simulink model "Robot"  (R2022b)
settings: Solver=FixedStepDiscrete  StartTime=0.0  StopTime=30  FixedStep=0.001  RelTol=1e-3
InitFcn:
  | load("BusConfig.mat");
undefined symbols (not defined in the file or in its folder): DiscIntNeverNeededParam
libraries: slrealtimeethercatlib x119, simulink x20
(part 3 of 7)

== system Robot/Motor2 Torque Control Init Frame/State_2_Enable ==
  State : Inport
  Subsystem : Subsystem
  Switch Case : SwitchCase  CaseConditions={TaskIndex}
  Enable : Outport
  FinishIndex : Outport  Port=2
  wires:
  Switch Case/2 -> Subsystem/2(Case Default)
  Switch Case/1 -> Subsystem/1(Case)
  Subsystem/2(FinishIndex) -> FinishIndex/1
  Subsystem/1(Enable) -> Enable/1
  State/1 -> Switch Case/1

== system Robot/Motor2 Torque Control Init Frame/State_3_Enable ==
  State : Inport
  Subsystem : Subsystem
  Switch Case : SwitchCase  CaseConditions={TaskIndex}
  Enable : Outport
  FinishIndex : Outport  Port=2
  wires:
  Switch Case/2 -> Subsystem/2(Case Default)
  Switch Case/1 -> Subsystem/1(Case)
  Subsystem/2(FinishIndex) -> FinishIndex/1
  Subsystem/1(Enable) -> Enable/1
  State/1 -> Switch Case/1

== system Robot/Motor2 Torque Control Init Frame/State_4_Enable ==
  State : Inport
  Subsystem : Subsystem
  Switch Case : SwitchCase  CaseConditions={TaskIndex}
  Enable : Outport
  FinishIndex : Outport  Port=2
  wires:
  Switch Case/2 -> Subsystem/2(Case Default)
  Switch Case/1 -> Subsystem/1(Case)
  Subsystem/2(FinishIndex) -> FinishIndex/1
  Subsystem/1(Enable) -> Enable/1
  State/1 -> Switch Case/1

== system Robot/Motor2 Torque Control Init Frame/State_5_Enable ==
  State : Inport
  Subsystem : Subsystem
  Switch Case : SwitchCase  CaseConditions={TaskIndex}
  Enable : Outport
  FinishIndex : Outport  Port=2
  wires:
  Switch Case/2 -> Subsystem/2(Case Default)
  Switch Case/1 -> Subsystem/1(Case)
  Subsystem/2(FinishIndex) -> FinishIndex/1
  Subsystem/1(Enable) -> Enable/1
  State/1 -> Switch Case/1

== system Robot/Motor2 Torque Control Init Frame/State_6_Enable ==
  State : Inport
  Subsystem : Subsystem
  Switch Case : SwitchCase  CaseConditions={TaskIndex}
  Enable : Outport
  FinishIndex : Outport  Port=2
  wires:
  Switch Case/2 -> Subsystem/2(Case Default)
  Switch Case/1 -> Subsystem/1(Case)
  Subsystem/2(FinishIndex) -> FinishIndex/1
  Subsystem/1(Enable) -> Enable/1
  State/1 -> Switch Case/1

== system Robot/Motor2 Torque Control Init Frame/State_7_Enable ==
  State : Inport
  Subsystem : Subsystem
  Switch Case : SwitchCase  CaseConditions={TaskIndex}
  Enable : Outport
  FinishIndex : Outport  Port=2
  wires:
  Switch Case/2 -> Subsystem/2(Case Default)
  Switch Case/1 -> Subsystem/1(Case)
  Subsystem/2(FinishIndex) -> FinishIndex/1
  Subsystem/1(Enable) -> Enable/1
  State/1 -> Switch Case/1

== system Robot/Motor2 Torque Control Init Frame/State_8_Enable ==
  State : Inport
  Subsystem : Subsystem
  Switch Case : SwitchCase  CaseConditions={TaskIndex}
  Enable : Outport
  FinishIndex : Outport  Port=2
  wires:
  Switch Case/2 -> Subsystem/2(Case Default)
  Switch Case/1 -> Subsystem/1(Case)
  Subsystem/2(FinishIndex) -> FinishIndex/1
  Subsystem/1(Enable) -> Enable/1
  State/1 -> Switch Case/1

== system Robot/Motor2 Torque Control Init Frame/State_9_Enable ==
  State : Inport
  Subsystem : Subsystem
  Switch Case : SwitchCase  CaseConditions={TaskIndex}
  Enable : Outport
  FinishIndex : Outport  Port=2
  wires:
  Switch Case/2 -> Subsystem/2(Case Default)
  Switch Case/1 -> Subsystem/1(Case)
  Subsystem/2(FinishIndex) -> FinishIndex/1
  Subsystem/1(Enable) -> Enable/1
  State/1 -> Switch Case/1

== system Robot/Motor3 Torque Control Init Frame/Get MasterState OP Frame ==
  FinishIndex : Inport
  Enable : EnablePort
  Clock : Clock
  Constant4 : Constant  Value=0  OutDataTypeStr=double
  Constant5 : Constant
  Display{1,3..5} (4 alike) : Display
  EtherCAT PDO Receive1 : slrealtimeethercatlib/EtherCAT PDO Receive  Priority=2  sig_name=Drive 3 (Elmo Drive ).Inputs.Status word  sig_offset=24832  sig_type=uint16  type_size=16  sig_dim=1  device_id=0  sample_time=0.001000
  Get Device State : slrealtimeethercatlib/Get Device State  device_id=0  slave_name=Drive 3 (Elmo Drive )  sample_time=0.001  slave_addr=1003  selected_slave=Term 1 (EK1100)  timeout=500  slave_found=1
  If Action Subsystem5 : Subsystem  TreatAsAtomicUnit=on
  If Action Subsystem6 : Subsystem  TreatAsAtomicUnit=on
  If Action Subsystem7 : Subsystem  TreatAsAtomicUnit=on
  If1 : If  IfExpression=(u1 == 4663)
  If2 : If  IfExpression=(u1 == 8)
  Merge1 : Merge
  TaskFinished : Outport
  wires:
  If Action Subsystem6/1(Out1) -> Merge1/2
  EtherCAT PDO Receive1/1 -> Display3/1
  Get Device State/1 -> If2/1, Display1/1
  If Action Subsystem7/1(Out1) -> Display5/1
  If Action Subsystem5/1(Out1) -> Merge1/1
  Constant4/1 -> If Action Subsystem6/1(In1)
  Merge1/1 -> TaskFinished/1
  If1/1 -> If Action Subsystem7/Action
  Constant5/1 -> If Action Subsystem7/1(In1)
  If2/1 -> If Action Subsystem5/Action
  If2/2 -> If Action Subsystem6/Action
  Clock/1 -> Display4/1
  FinishIndex/1 -> If Action Subsystem5/1(In1)

== system Robot/Motor3 Torque Control Init Frame/PDO Set 0x6040:6->7->15 Frame ==
  FinishIndex : Inport
  Enable : EnablePort
  Clock : Clock
  Constant : Constant  Value=6  OutDataTypeStr=uint16
  Constant1 : Constant  Value=7  OutDataTypeStr=uint16
  Constant2 : Constant  Value=15  OutDataTypeStr=uint16
  Constant4 : Constant  Value=0  OutDataTypeStr=double
  Constant5 : Constant
  Counter Limited : simulink/Sources/Counter Limited  uplimit=500  tsamp=-1
  Display{1..5} (5 alike) : Display
  EtherCAT PDO Receive1 : slrealtimeethercatlib/EtherCAT PDO Receive  Priority=2  sig_name=Drive 3 (Elmo Drive ).Inputs.Status word  sig_offset=24832  sig_type=uint16  type_size=16  sig_dim=1  device_id=0  sample_time=0.001000
  EtherCAT PDO Transmit1 : slrealtimeethercatlib/EtherCAT PDO Transmit  Priority=3  sig_name=Drive 3 (Elmo Drive ).Outputs.Control word  sig_offset=24800  sig_type=uint16  type_size=16  sig_dim=1  device_id=0  sample_time=0.001000
  If : If  NumInputs=2  IfExpression=(u1 == 720)&(u2 == 500)  ElseIfExpressions=(u1 == 689)&(u2 == 500), (u1 == 691)&(u2 == 500)
  If Action Subsystem : Subsystem  TreatAsAtomicUnit=on
  If Action Subsystem1 : Subsystem  TreatAsAtomicUnit=on
  If Action Subsystem2 : Subsystem  TreatAsAtomicUnit=on
  If Action Subsystem4 : Subsystem  TreatAsAtomicUnit=on
  If Action Subsystem5 : Subsystem  TreatAsAtomicUnit=on
  If Action Subsystem6 : Subsystem  TreatAsAtomicUnit=on
  If Action Subsystem7 : Subsystem  TreatAsAtomicUnit=on
  If1 : If  IfExpression=(u1 == 4663)|(u1 == 4791)
  If2 : If  IfExpression=(u1 >= 0.1)
  Memory : Memory
  Merge : Merge  Inputs=4
  Merge1 : Merge
  TaskFinished : Outport
  wires:
  If Action Subsystem2/1(Out1) -> Merge/3
  If Action Subsystem7/1(Out1) -> If2/1, Display5/1
  If Action Subsystem6/1(Out1) -> Merge1/2
  EtherCAT PDO Receive1/1 -> If1/1, If/1, Display1/1
  If/2 -> If Action Subsystem1/Action
  Memory/1 -> If Action Subsystem4/1(In1)
  Constant5/1 -> If Action Subsystem7/1(In1)
  Constant1/1 -> If Action Subsystem1/1(In1)
  Constant/1 -> If Action Subsystem/1(In1)
  If Action Subsystem1/1(Out1) -> Merge/2
  If/4 -> If Action Subsystem4/Action
  Constant2/1 -> If Action Subsystem2/1(In1)
  If/3 -> If Action Subsystem2/Action
  If/1 -> If Action Subsystem/Action
  Clock/1 -> Display4/1
  If1/1 -> If Action Subsystem7/Action
  If2/1 -> If Action Subsystem5/Action
  Merge/1 -> Display2/1, EtherCAT PDO Transmit1/1, Memory/1
  Merge1/1 -> TaskFinished/1
  FinishIndex/1 -> If Action Subsystem5/1(In1)
  If2/2 -> If Action Subsystem6/Action
  If Action Subsystem4/1(Out1) -> Merge/4
  Counter Limited/1 -> If/2, Display3/1
  Constant4/1 -> If Action Subsystem6/1(In1)
  If Action Subsystem5/1(Out1) -> Merge1/1
  If Action Subsystem/1(Out1) -> Merge/1

== system Robot/Motor3 Torque Control Init Frame/SDO Get 0x6075 Frame ==
  FinishIndex : Inport
  Enable : EnablePort
  Clock : Clock
  Constant : Constant  OutDataTypeStr=int32
  Constant4 : Constant  Value=0  OutDataTypeStr=double
  Constant5 : Constant
  Display{,1,3..5} (5 alike) : Display
  EtherCAT Async SDO Upload : slrealtimeethercatlib/EtherCAT Async SDO Upload  index=0x6075  subIndex=0  sig_type=uint32  sig_dim=1  device_id=0  slave_name=Drive 3 (Elmo Drive )  sample_time=-1  slave_addr=1003  selected_slave=Term 1 (EK1100)  timeout=3000  slave_found=1  complete=0
  If Action Subsystem5 : Subsystem  TreatAsAtomicUnit=on
  If Action Subsystem6 : Subsystem  TreatAsAtomicUnit=on
  If Action Subsystem7 : Subsystem  TreatAsAtomicUnit=on
  If1 : If  IfExpression=(u1 == 4663)
  If2 : If  IfExpression=(u1 == 2)
  Merge1 : Merge
  TaskFinished : Outport
  RatedCurrent : Outport  Port=2
  wires:
  EtherCAT Async SDO Upload/1 -> RatedCurrent/1, Display/1
  EtherCAT Async SDO Upload/3 -> Display3/1
  EtherCAT Async SDO Upload/2 -> If2/1, Display1/1
  Constant/1 -> EtherCAT Async SDO Upload/1
  If2/1 -> If Action Subsystem5/Action
  Merge1/1 -> TaskFinished/1
  Clock/1 -> Display4/1
  If2/2 -> If Action Subsystem6/Action
  If Action Subsystem7/1(Out1) -> Display5/1
  Constant4/1 -> If Action Subsystem6/1(In1)
  If1/1 -> If Action Subsystem7/Action
  If Action Subsystem5/1(Out1) -> Merge1/1
  If Action Subsystem6/1(Out1) -> Merge1/2
  Constant5/1 -> If Action Subsystem7/1(In1)
  FinishIndex/1 -> If Action Subsystem5/1(In1)

== system Robot/Motor3 Torque Control Init Frame/SDO Set 0x6040:15 Frame ==
  FinishIndex : Inport
  Enable : EnablePort
  Bitwise Operator : simulink/Logic and Bit Operations/Bitwise Operator  logicop=AND  UseBitMask=on  BitMask=bin2dec('0000000000000111')  BitMaskRealWorld=Stored Integer
  Clock : Clock
  Constant : Constant  Value=15  OutDataTypeStr=uint16
  Constant1 : Constant  OutDataTypeStr=int32
  Constant2 : Constant  Value=0  OutDataTypeStr=int32
  Constant4 : Constant  Value=0  OutDataTypeStr=double
  Constant5 : Constant
  Constant6 : Constant  OutDataTypeStr=int32
  Constant7 : Constant
  Constant8 : Constant  Value=0b0000000000000111  OutDataTypeStr=uint16
  Display{1..6} (6 alike) : Display
  EtherCAT Async SDO Download : slrealtimeethercatlib/EtherCAT Async SDO Download  index=0x6040  subIndex=0  sig_type=uint16  sig_dim=1  device_id=0  slave_name=Drive 3 (Elmo Drive )  sample_time=-1  slave_addr=1003  selected_slave=Term 1 (EK1100)  timeout=2000  slave_found=1  complete=0
  EtherCAT PDO Receive1 : slrealtimeethercatlib/EtherCAT PDO Receive  Priority=2  sig_name=Drive 4 (Elmo Drive ).Inputs.Status word  sig_offset=39136  sig_type=uint16  type_size=16  sig_dim=1  device_id=0  sample_time=0.001
  If Action Subsystem1 : Subsystem  TreatAsAtomicUnit=on
  If Action Subsystem2 : Subsystem  TreatAsAtomicUnit=on
  If Action Subsystem3 : Subsystem  TreatAsAtomicUnit=on
  If Action Subsystem5 : Subsystem  TreatAsAtomicUnit=on
  If Action Subsystem6 : Subsystem  TreatAsAtomicUnit=on
  If Action Subsystem7 : Subsystem  TreatAsAtomicUnit=on
  If1 : If  IfExpression=(u1 == 4663)
  If2 : If  IfExpression=(u1 == 2)
  If3 : If  NumInputs=2  IfExpression=(u1 == u2)
  If4 : If  IfExpression=(u1 >= 0.1)
  Merge1 : Merge
  Merge2 : Merge
  TaskFinished : Outport
  wires:
  Constant8/1 -> If3/2
  Bitwise Operator/1 -> If3/1
  If Action Subsystem3/1(Out1) -> Display6/1, If4/1
  Clock/1 -> Display4/1
  Merge1/1 -> TaskFinished/1
  If Action Subsystem2/1(Out1) -> Merge2/2
  If Action Subsystem1/1(Out1) -> Merge2/1
  Constant7/1 -> If Action Subsystem3/1(In1)
  If2/2 -> If Action Subsystem6/Action
  EtherCAT PDO Receive1/1 -> Display3/1, Bitwise Operator/1
  If3/1 -> If Action Subsystem3/Action
  If4/1 -> If Action Subsystem1/Action
  Constant6/1 -> If Action Subsystem2/1(In1)
  If4/2 -> If Action Subsystem2/Action
  EtherCAT Async SDO Download/1 -> If2/1, Display1/1
  Constant4/1 -> If Action Subsystem6/1(In1)
  Constant5/1 -> If Action Subsystem7/1(In1)
  Constant1/1 -> EtherCAT Async SDO Download/2
  If Action Subsystem6/1(Out1) -> Merge1/2
  If Action Subsystem7/1(Out1) -> Display5/1
  If2/1 -> If Action Subsystem5/Action
  Constant2/1 -> If Action Subsystem1/1(In1)
  If1/1 -> If Action Subsystem7/Action
  FinishIndex/1 -> If Action Subsystem5/1(In1)
  EtherCAT Async SDO Download/2 -> Display2/1
  Constant/1 -> EtherCAT Async SDO Download/1
  If Action Subsystem5/1(Out1) -> Merge1/1

== system Robot/Motor3 Torque Control Init Frame/SDO Set 0x6040:31 Frame ==
  FinishIndex : Inport
  Enable : EnablePort
  Bitwise Operator : simulink/Logic and Bit Operations/Bitwise Operator  logicop=AND  UseBitMask=on  BitMask=bin2dec('0001010000010111')  BitMaskRealWorld=Stored Integer
  Clock : Clock
  Constant : Constant  Value=31  OutDataTypeStr=uint16
  Constant1 : Constant  OutDataTypeStr=int32
  Constant2 : Constant  Value=0  OutDataTypeStr=int32
  Constant4 : Constant  Value=0  OutDataTypeStr=double
  Constant5 : Constant
  Constant6 : Constant  OutDataTypeStr=int32
  Constant7 : Constant
  Constant8 : Constant  Value=0b0001010000010111  OutDataTypeStr=uint16
  Display{1..6} (6 alike) : Display
  EtherCAT Async SDO Download : slrealtimeethercatlib/EtherCAT Async SDO Download  index=0x6040  subIndex=0  sig_type=uint16  sig_dim=1  device_id=0  slave_name=Drive 3 (Elmo Drive )  sample_time=-1  slave_addr=1003  selected_slave=Term 1 (EK1100)  timeout=2000  slave_found=1  complete=0
  EtherCAT PDO Receive1 : slrealtimeethercatlib/EtherCAT PDO Receive  Priority=2  sig_name=Drive 3 (Elmo Drive ).Inputs.Status word  sig_offset=24832  sig_type=uint16  type_size=16  sig_dim=1  device_id=0  sample_time=0.001
  If Action Subsystem1 : Subsystem  TreatAsAtomicUnit=on
  If Action Subsystem2 : Subsystem  TreatAsAtomicUnit=on
  If Action Subsystem3 : Subsystem  TreatAsAtomicUnit=on
  If Action Subsystem5 : Subsystem  TreatAsAtomicUnit=on
  If Action Subsystem6 : Subsystem  TreatAsAtomicUnit=on
  If Action Subsystem7 : Subsystem  TreatAsAtomicUnit=on
  If1 : If  IfExpression=(u1 == 4663)
  If2 : If  IfExpression=(u1 == 2)
  If3 : If  NumInputs=2  IfExpression=(u1 == u2)
  If4 : If  IfExpression=(u1 >= 0.1)
  Merge1 : Merge
  Merge2 : Merge
  TaskFinished : Outport
  wires:
  If1/1 -> If Action Subsystem7/Action
  If Action Subsystem5/1(Out1) -> Merge1/1
  If Action Subsystem6/1(Out1) -> Merge1/2
  FinishIndex/1 -> If Action Subsystem5/1(In1)
  If2/1 -> If Action Subsystem5/Action
  If4/2 -> If Action Subsystem2/Action
  EtherCAT Async SDO Download/1 -> If2/1, Display1/1
  Constant/1 -> EtherCAT Async SDO Download/1
  Bitwise Operator/1 -> If3/1
  If Action Subsystem7/1(Out1) -> Display5/1
  Constant8/1 -> If3/2
  If2/2 -> If Action Subsystem6/Action
  If Action Subsystem3/1(Out1) -> Display6/1, If4/1
  If Action Subsystem2/1(Out1) -> Merge2/2
  If3/1 -> If Action Subsystem3/Action
  Constant4/1 -> If Action Subsystem6/1(In1)
  Constant6/1 -> If Action Subsystem2/1(In1)
  If4/1 -> If Action Subsystem1/Action
  Constant1/1 -> EtherCAT Async SDO Download/2
  EtherCAT PDO Receive1/1 -> Display3/1, Bitwise Operator/1
  Clock/1 -> Display4/1
  If Action Subsystem1/1(Out1) -> Merge2/1
  Merge1/1 -> TaskFinished/1
  Constant2/1 -> If Action Subsystem1/1(In1)
  EtherCAT Async SDO Download/2 -> Display2/1
  Constant5/1 -> If Action Subsystem7/1(In1)
  Constant7/1 -> If Action Subsystem3/1(In1)

== system Robot/Motor3 Torque Control Init Frame/SDO Set 0x6040:6 Frame ==
  FinishIndex : Inport
  Enable : EnablePort
  Bitwise Operator : simulink/Logic and Bit Operations/Bitwise Operator  logicop=AND  UseBitMask=on  BitMask=bin2dec('0000000000000001')  BitMaskRealWorld=Stored Integer
  Clock : Clock
  Constant : Constant  Value=6  OutDataTypeStr=uint16
  Constant1 : Constant  OutDataTypeStr=int32
  Constant2 : Constant  Value=0  OutDataTypeStr=int32
  Constant4 : Constant  Value=0  OutDataTypeStr=double
  Constant5 : Constant
  Constant6 : Constant  OutDataTypeStr=int32
  Constant7 : Constant
  Constant8 : Constant  Value=0b0000000000000001  OutDataTypeStr=uint16
  Display{1..6} (6 alike) : Display
  EtherCAT Async SDO Download : slrealtimeethercatlib/EtherCAT Async SDO Download  index=0x6040  subIndex=0  sig_type=uint16  sig_dim=1  device_id=0  slave_name=Drive 3 (Elmo Drive )  sample_time=-1  slave_addr=1003  selected_slave=Term 1 (EK1100)  timeout=3000  slave_found=1  complete=0
  EtherCAT PDO Receive1 : slrealtimeethercatlib/EtherCAT PDO Receive  Priority=2  sig_name=Drive 3 (Elmo Drive ).Inputs.Status word  sig_offset=24832  sig_type=uint16  type_size=16  sig_dim=1  device_id=0  sample_time=0.001
  If Action Subsystem1 : Subsystem  TreatAsAtomicUnit=on
  If Action Subsystem2 : Subsystem  TreatAsAtomicUnit=on
  If Action Subsystem3 : Subsystem  TreatAsAtomicUnit=on
  If Action Subsystem5 : Subsystem  TreatAsAtomicUnit=on
  If Action Subsystem6 : Subsystem  TreatAsAtomicUnit=on
  If Action Subsystem7 : Subsystem  TreatAsAtomicUnit=on
  If1 : If  IfExpression=(u1 == 4663)
  If2 : If  IfExpression=(u1 == 2)
  If3 : If  NumInputs=2  IfExpression=(u1 == u2)
  If4 : If  IfExpression=(u1 >= 0.1)
  Merge1 : Merge
  Merge2 : Merge
  TaskFinished : Outport
  wires:
  Constant2/1 -> If Action Subsystem1/1(In1)
  Constant/1 -> EtherCAT Async SDO Download/1
  If1/1 -> If Action Subsystem7/Action
  Constant4/1 -> If Action Subsystem6/1(In1)
  If4/1 -> If Action Subsystem1/Action
  If Action Subsystem1/1(Out1) -> Merge2/1
  If2/2 -> If Action Subsystem6/Action
  Bitwise Operator/1 -> If3/1
  FinishIndex/1 -> If Action Subsystem5/1(In1)
  EtherCAT Async SDO Download/2 -> Display2/1
  EtherCAT Async SDO Download/1 -> If2/1, Display1/1
  If2/1 -> If Action Subsystem5/Action
  If4/2 -> If Action Subsystem2/Action
  Constant5/1 -> If Action Subsystem7/1(In1)
  If Action Subsystem2/1(Out1) -> Merge2/2
  Constant7/1 -> If Action Subsystem3/1(In1)
  If Action Subsystem3/1(Out1) -> Display6/1, If4/1
  If Action Subsystem5/1(Out1) -> Merge1/1
  Constant6/1 -> If Action Subsystem2/1(In1)
  If Action Subsystem6/1(Out1) -> Merge1/2
  Constant1/1 -> EtherCAT Async SDO Download/2
  If3/1 -> If Action Subsystem3/Action
  If Action Subsystem7/1(Out1) -> Display5/1
  Constant8/1 -> If3/2
  EtherCAT PDO Receive1/1 -> Display3/1, Bitwise Operator/1
  Clock/1 -> Display4/1
  Merge1/1 -> TaskFinished/1

== system Robot/Motor3 Torque Control Init Frame/SDO Set 0x6040:7 Frame ==
  FinishIndex : Inport
  Enable : EnablePort
  Bitwise Operator : simulink/Logic and Bit Operations/Bitwise Operator  logicop=AND  UseBitMask=on  BitMask=bin2dec('0000000000000011')  BitMaskRealWorld=Stored Integer
  Clock : Clock
  Constant : Constant  Value=7  OutDataTypeStr=uint16
  Constant1 : Constant  OutDataTypeStr=int32
  Constant2 : Constant  Value=0  OutDataTypeStr=int32
  Constant4 : Constant  Value=0  OutDataTypeStr=double
  Constant5 : Constant
  Constant6 : Constant  OutDataTypeStr=int32
  Constant7 : Constant
  Constant8 : Constant  Value=0b0000000000000011  OutDataTypeStr=uint16
  Display{1..6} (6 alike) : Display
  EtherCAT Async SDO Download : slrealtimeethercatlib/EtherCAT Async SDO Download  index=0x6040  subIndex=0  sig_type=uint16  sig_dim=1  device_id=0  slave_name=Drive 3 (Elmo Drive )  sample_time=-1  slave_addr=1003  selected_slave=Term 1 (EK1100)  timeout=2000  slave_found=1  complete=0
  EtherCAT PDO Receive1 : slrealtimeethercatlib/EtherCAT PDO Receive  Priority=2  sig_name=Drive 3 (Elmo Drive ).Inputs.Status word  sig_offset=24832  sig_type=uint16  type_size=16  sig_dim=1  device_id=0  sample_time=0.001
  If Action Subsystem1 : Subsystem  TreatAsAtomicUnit=on
  If Action Subsystem2 : Subsystem  TreatAsAtomicUnit=on
  If Action Subsystem3 : Subsystem  TreatAsAtomicUnit=on
  If Action Subsystem5 : Subsystem  TreatAsAtomicUnit=on
  If Action Subsystem6 : Subsystem  TreatAsAtomicUnit=on
  If Action Subsystem7 : Subsystem  TreatAsAtomicUnit=on
  If1 : If  IfExpression=(u1 == 4663)
  If2 : If  IfExpression=(u1 == 2)
  If3 : If  NumInputs=2  IfExpression=(u1 == u2)
  If4 : If  IfExpression=(u1 >= 0.1)
  Merge1 : Merge
  Merge2 : Merge
  TaskFinished : Outport
  wires:
  EtherCAT PDO Receive1/1 -> Display3/1, Bitwise Operator/1
  Constant1/1 -> EtherCAT Async SDO Download/2
  Constant/1 -> EtherCAT Async SDO Download/1
  If Action Subsystem1/1(Out1) -> Merge2/1
  Constant7/1 -> If Action Subsystem3/1(In1)
  EtherCAT Async SDO Download/2 -> Display2/1
  Constant4/1 -> If Action Subsystem6/1(In1)
  FinishIndex/1 -> If Action Subsystem5/1(In1)
  If Action Subsystem6/1(Out1) -> Merge1/2
  Constant2/1 -> If Action Subsystem1/1(In1)
  If Action Subsystem5/1(Out1) -> Merge1/1
  Constant5/1 -> If Action Subsystem7/1(In1)
  If4/2 -> If Action Subsystem2/Action
  If2/1 -> If Action Subsystem5/Action
  If Action Subsystem7/1(Out1) -> Display5/1
  Merge1/1 -> TaskFinished/1
  Constant6/1 -> If Action Subsystem2/1(In1)
  Bitwise Operator/1 -> If3/1
  If Action Subsystem3/1(Out1) -> Display6/1, If4/1
  If1/1 -> If Action Subsystem7/Action
  If4/1 -> If Action Subsystem1/Action
  Clock/1 -> Display4/1
  If3/1 -> If Action Subsystem3/Action
  If Action Subsystem2/1(Out1) -> Merge2/2
  Constant8/1 -> If3/2
  If2/2 -> If Action Subsystem6/Action
  EtherCAT Async SDO Download/1 -> If2/1, Display1/1

== system Robot/Motor3 Torque Control Init Frame/SDO Set 0x6060:10 Frame ==
  FinishIndex : Inport
  Enable : EnablePort
  Clock : Clock
  Constant : Constant  Value=10  OutDataTypeStr=int8
  Constant1 : Constant  OutDataTypeStr=int32
  Constant4 : Constant  Value=0  OutDataTypeStr=double
  Constant5 : Constant
  Display{1..2,4..5} (4 alike) : Display
  EtherCAT Async SDO Download : slrealtimeethercatlib/EtherCAT Async SDO Download  index=0x6060  subIndex=0  sig_type=int8  sig_dim=1  device_id=0  slave_name=Drive 3 (Elmo Drive )  sample_time=-1  slave_addr=1003  selected_slave=Term 1 (EK1100)  timeout=2000  slave_found=1  complete=0
  If Action Subsystem5 : Subsystem  TreatAsAtomicUnit=on
  If Action Subsystem6 : Subsystem  TreatAsAtomicUnit=on
  If Action Subsystem7 : Subsystem  TreatAsAtomicUnit=on
  If1 : If  IfExpression=(u1 == 4663)
  If2 : If  IfExpression=(u1 == 2)
  Merge1 : Merge
  TaskFinished : Outport
  wires:
  EtherCAT Async SDO Download/2 -> Display2/1
  If Action Subsystem7/1(Out1) -> Display5/1
  If Action Subsystem6/1(Out1) -> Merge1/2
  If2/1 -> If Action Subsystem5/Action
  If2/2 -> If Action Subsystem6/Action
  Constant/1 -> EtherCAT Async SDO Download/1
  If1/1 -> If Action Subsystem7/Action
  Merge1/1 -> TaskFinished/1
  If Action Subsystem5/1(Out1) -> Merge1/1
  Constant5/1 -> If Action Subsystem7/1(In1)
  Clock/1 -> Display4/1
  Constant1/1 -> EtherCAT Async SDO Download/2
  Constant4/1 -> If Action Subsystem6/1(In1)
  FinishIndex/1 -> If Action Subsystem5/1(In1)
  EtherCAT Async SDO Download/1 -> If2/1, Display1/1

== system Robot/Motor3 Torque Control Init Frame/SDO Set 0x6060:6 Frame ==
  FinishIndex : Inport
  Enable : EnablePort
  Clock : Clock
  Constant : Constant  Value=6  OutDataTypeStr=int8
  Constant1 : Constant  OutDataTypeStr=int32
  Constant4 : Constant  Value=0  OutDataTypeStr=double
  Constant5 : Constant
  Display{1..2,4..5} (4 alike) : Display
  EtherCAT Async SDO Download : slrealtimeethercatlib/EtherCAT Async SDO Download  index=0x6060  subIndex=0  sig_type=int8  sig_dim=1  device_id=0  slave_name=Drive 3 (Elmo Drive )  sample_time=-1  slave_addr=1003  selected_slave=Term 1 (EK1100)  timeout=2000  slave_found=1  complete=0
  If Action Subsystem5 : Subsystem  TreatAsAtomicUnit=on
  If Action Subsystem6 : Subsystem  TreatAsAtomicUnit=on
  If Action Subsystem7 : Subsystem  TreatAsAtomicUnit=on
  If1 : If  IfExpression=(u1 == 4663)
  If2 : If  IfExpression=(u1 == 2)
  Merge1 : Merge
  TaskFinished : Outport
  wires:
  FinishIndex/1 -> If Action Subsystem5/1(In1)
  If2/1 -> If Action Subsystem5/Action
  If Action Subsystem5/1(Out1) -> Merge1/1
  If Action Subsystem6/1(Out1) -> Merge1/2
  EtherCAT Async SDO Download/2 -> Display2/1
  If2/2 -> If Action Subsystem6/Action
  Constant1/1 -> EtherCAT Async SDO Download/2
  Merge1/1 -> TaskFinished/1
  If Action Subsystem7/1(Out1) -> Display5/1
  Clock/1 -> Display4/1
  EtherCAT Async SDO Download/1 -> If2/1, Display1/1
  Constant4/1 -> If Action Subsystem6/1(In1)
  Constant5/1 -> If Action Subsystem7/1(In1)
  If1/1 -> If Action Subsystem7/Action
  Constant/1 -> EtherCAT Async SDO Download/1

== system Robot/Motor3 Torque Control Init Frame/SDO Set 0x6080:-1 Frame ==
  FinishIndex : Inport
  Enable : EnablePort
  Clock : Clock
  Constant : Constant  Value=(2^31)-1  OutDataTypeStr=int32
  Constant1 : Constant  OutDataTypeStr=int32
  Constant4 : Constant  Value=0  OutDataTypeStr=double
  Constant5 : Constant
  Display{1..2,4..5} (4 alike) : Display
  EtherCAT Async SDO Download : slrealtimeethercatlib/EtherCAT Async SDO Download  index=0x6080  subIndex=0  sig_type=int32  sig_dim=1  device_id=0  slave_name=Drive 3 (Elmo Drive )  sample_time=-1  slave_addr=1003  selected_slave=Term 1 (EK1100)  timeout=3000  slave_found=1  complete=0
  If Action Subsystem5 : Subsystem  TreatAsAtomicUnit=on
  If Action Subsystem6 : Subsystem  TreatAsAtomicUnit=on
  If Action Subsystem7 : Subsystem  TreatAsAtomicUnit=on
  If1 : If  IfExpression=(u1 == 4663)
  If2 : If  IfExpression=(u1 == 2)
  Merge1 : Merge
  TaskFinished : Outport
  wires:
  Merge1/1 -> TaskFinished/1
  EtherCAT Async SDO Download/1 -> If2/1, Display1/1
  EtherCAT Async SDO Download/2 -> Display2/1
  Constant1/1 -> EtherCAT Async SDO Download/2
  FinishIndex/1 -> If Action Subsystem5/1(In1)
  If2/2 -> If Action Subsystem6/Action
  If2/1 -> If Action Subsystem5/Action
  Constant4/1 -> If Action Subsystem6/1(In1)
  Constant/1 -> EtherCAT Async SDO Download/1
  Constant5/1 -> If Action Subsystem7/1(In1)
  Clock/1 -> Display4/1
  If1/1 -> If Action Subsystem7/Action
  If Action Subsystem7/1(Out1) -> Display5/1
  If Action Subsystem6/1(Out1) -> Merge1/2
  If Action Subsystem5/1(Out1) -> Merge1/1

== system Robot/Motor3 Torque Control Init Frame/SDO Set 0x6098:35 Frame ==
  FinishIndex : Inport
  Enable : EnablePort
  Clock : Clock
  Constant : Constant  Value=35  OutDataTypeStr=int8
  Constant1 : Constant  OutDataTypeStr=int32
  Constant4 : Constant  Value=0  OutDataTypeStr=double
  Constant5 : Constant
  Display{1..2,4..5} (4 alike) : Display
  EtherCAT Async SDO Download : slrealtimeethercatlib/EtherCAT Async SDO Download  index=0x6098  subIndex=0  sig_type=int8  sig_dim=1  device_id=0  slave_name=Drive 3 (Elmo Drive )  sample_time=-1  slave_addr=1003  selected_slave=Term 1 (EK1100)  timeout=2000  slave_found=1  complete=0
  If Action Subsystem5 : Subsystem  TreatAsAtomicUnit=on
  If Action Subsystem6 : Subsystem  TreatAsAtomicUnit=on
  If Action Subsystem7 : Subsystem  TreatAsAtomicUnit=on
  If1 : If  IfExpression=(u1 == 4663)
  If2 : If  IfExpression=(u1 == 2)
  Merge1 : Merge
  TaskFinished : Outport
  wires:
  EtherCAT Async SDO Download/2 -> Display2/1
  EtherCAT Async SDO Download/1 -> If2/1, Display1/1
  Constant1/1 -> EtherCAT Async SDO Download/2
  FinishIndex/1 -> If Action Subsystem5/1(In1)
  Constant4/1 -> If Action Subsystem6/1(In1)
  If Action Subsystem5/1(Out1) -> Merge1/1
  Constant5/1 -> If Action Subsystem7/1(In1)
  Merge1/1 -> TaskFinished/1
  If2/1 -> If Action Subsystem5/Action
  If Action Subsystem7/1(Out1) -> Display5/1
  Constant/1 -> EtherCAT Async SDO Download/1
  If2/2 -> If Action Subsystem6/Action
  If Action Subsystem6/1(Out1) -> Merge1/2
  If1/1 -> If Action Subsystem7/Action
  Clock/1 -> Display4/1

== system Robot/Motor3 Torque Control Init Frame/Set MasterState to OP Frame ==
  FinishIndex : Inport
  Enable : EnablePort
  Clock : Clock
  Constant1 : Constant  OutDataTypeStr=boolean
  Constant2 : Constant  Value=8  OutDataTypeStr=int32
  Constant4 : Constant  Value=0  OutDataTypeStr=double
  Constant5 : Constant
  Display{1..2,4..5} (4 alike) : Display
  If Action Subsystem5 : Subsystem  TreatAsAtomicUnit=on
  If Action Subsystem6 : Subsystem  TreatAsAtomicUnit=on
  If Action Subsystem7 : Subsystem  TreatAsAtomicUnit=on
  If1 : If  IfExpression=(u1 == 8)
  If2 : If  IfExpression=(u1 > 0.1)
  Merge1 : Merge
  Set Device State : slrealtimeethercatlib/Set Device State  device_id=0  slave_name=Drive 3 (Elmo Drive )  sample_time=-1  slave_addr=1003  selected_slave=Term 1 (EK1100)  slave_found=1
  TaskFinished : Outport
  wires:
  Set Device State/1 -> If1/1, Display1/1
  Merge1/1 -> TaskFinished/1
  Constant1/1 -> Set Device State/2
  Constant4/1 -> If Action Subsystem6/1(In1)
  If1/1 -> If Action Subsystem7/Action
  FinishIndex/1 -> If Action Subsystem5/1(In1)
  Clock/1 -> Display4/1
  Set Device State/2 -> Display2/1
  If Action Subsystem5/1(Out1) -> Merge1/1
  If2/2 -> If Action Subsystem6/Action
  If2/1 -> If Action Subsystem5/Action
  If Action Subsystem7/1(Out1) -> If2/1, Display5/1
  If Action Subsystem6/1(Out1) -> Merge1/2
  Constant2/1 -> Set Device State/1
  Constant5/1 -> If Action Subsystem7/1(In1)

== system Robot/Motor3 Torque Control Init Frame/Set MasterState to SafeOP Frame ==
  FinishIndex : Inport
  Enable : EnablePort
  Clock : Clock
  Constant1 : Constant  OutDataTypeStr=boolean
  Constant2 : Constant  Value=4  OutDataTypeStr=int32
  Constant4 : Constant  Value=0  OutDataTypeStr=double
  Constant5 : Constant
  Display{1..2,4..5} (4 alike) : Display
  If Action Subsystem5 : Subsystem  TreatAsAtomicUnit=on
  If Action Subsystem6 : Subsystem  TreatAsAtomicUnit=on
  If Action Subsystem7 : Subsystem  TreatAsAtomicUnit=on
  If1 : If  IfExpression=(u1 == 4)
  If2 : If  IfExpression=(u1 > 0.1)
  Merge1 : Merge
  Set Device State : slrealtimeethercatlib/Set Device State  device_id=0  slave_name=Drive 3 (Elmo Drive )  sample_time=-1  slave_addr=1003  selected_slave=Term 1 (EK1100)  slave_found=1
  TaskFinished : Outport
  wires:
  Merge1/1 -> TaskFinished/1
  Set Device State/1 -> If1/1, Display1/1
  Constant1/1 -> Set Device State/2
  Constant2/1 -> Set Device State/1
  If Action Subsystem7/1(Out1) -> If2/1, Display5/1
  Constant5/1 -> If Action Subsystem7/1(In1)
  Clock/1 -> Display4/1
  If1/1 -> If Action Subsystem7/Action
  If2/1 -> If Action Subsystem5/Action
  If2/2 -> If Action Subsystem6/Action
  Set Device State/2 -> Display2/1
  If Action Subsystem6/1(Out1) -> Merge1/2
  Constant4/1 -> If Action Subsystem6/1(In1)
  FinishIndex/1 -> If Action Subsystem5/1(In1)
  If Action Subsystem5/1(Out1) -> Merge1/1

== system Robot/Motor3 Torque Control Init Frame/State_10_Enable ==
  State : Inport
  Subsystem : Subsystem
  Switch Case : SwitchCase  CaseConditions={TaskIndex}
  Enable : Outport
  FinishIndex : Outport  Port=2
  wires:
  Switch Case/2 -> Subsystem/2(Case Default)
  Switch Case/1 -> Subsystem/1(Case)
  Subsystem/2(FinishIndex) -> FinishIndex/1
  Subsystem/1(Enable) -> Enable/1
  State/1 -> Switch Case/1

== system Robot/Motor3 Torque Control Init Frame/State_11_Enable ==
  State : Inport
  Subsystem : Subsystem
  Switch Case : SwitchCase  CaseConditions={TaskIndex}
  Enable : Outport
  FinishIndex : Outport  Port=2
  wires:
  Switch Case/2 -> Subsystem/2(Case Default)
  Switch Case/1 -> Subsystem/1(Case)
  Subsystem/2(FinishIndex) -> FinishIndex/1
  Subsystem/1(Enable) -> Enable/1
  State/1 -> Switch Case/1

== system Robot/Motor3 Torque Control Init Frame/State_12_Enable ==
  State : Inport
  Subsystem : Subsystem
  Switch Case : SwitchCase  CaseConditions={TaskIndex}
  Enable : Outport
  FinishIndex : Outport  Port=2
  wires:
  Switch Case/2 -> Subsystem/2(Case Default)
  Switch Case/1 -> Subsystem/1(Case)
  Subsystem/2(FinishIndex) -> FinishIndex/1
  Subsystem/1(Enable) -> Enable/1
  State/1 -> Switch Case/1

== system Robot/Motor3 Torque Control Init Frame/State_13_Enable ==
  State : Inport
  Subsystem : Subsystem
  Switch Case : SwitchCase  CaseConditions={TaskIndex}
  Enable : Outport
  FinishIndex : Outport  Port=2
  wires:
  Switch Case/2 -> Subsystem/2(Case Default)
  Switch Case/1 -> Subsystem/1(Case)
  Subsystem/2(FinishIndex) -> FinishIndex/1
  Subsystem/1(Enable) -> Enable/1
  State/1 -> Switch Case/1

== system Robot/Motor3 Torque Control Init Frame/State_1_Enable ==
  State : Inport
  Subsystem : Subsystem
  Switch Case : SwitchCase  CaseConditions={TaskIndex}
  Enable : Outport
  FinishIndex : Outport  Port=2
  wires:
  Switch Case/2 -> Subsystem/2(Case Default)
  Switch Case/1 -> Subsystem/1(Case)
  Subsystem/2(FinishIndex) -> FinishIndex/1
  Subsystem/1(Enable) -> Enable/1
  State/1 -> Switch Case/1

== system Robot/Motor3 Torque Control Init Frame/State_2_Enable ==
  State : Inport
  Subsystem : Subsystem
  Switch Case : SwitchCase  CaseConditions={TaskIndex}
  Enable : Outport
  FinishIndex : Outport  Port=2
  wires:
  Switch Case/2 -> Subsystem/2(Case Default)
  Switch Case/1 -> Subsystem/1(Case)
  Subsystem/2(FinishIndex) -> FinishIndex/1
  Subsystem/1(Enable) -> Enable/1
  State/1 -> Switch Case/1

== system Robot/Motor3 Torque Control Init Frame/State_3_Enable ==
  State : Inport
  Subsystem : Subsystem
  Switch Case : SwitchCase  CaseConditions={TaskIndex}
  Enable : Outport
  FinishIndex : Outport  Port=2
  wires:
  Switch Case/2 -> Subsystem/2(Case Default)
  Switch Case/1 -> Subsystem/1(Case)
  Subsystem/2(FinishIndex) -> FinishIndex/1
  Subsystem/1(Enable) -> Enable/1
  State/1 -> Switch Case/1

== system Robot/Motor3 Torque Control Init Frame/State_4_Enable ==
  State : Inport
  Subsystem : Subsystem
  Switch Case : SwitchCase  CaseConditions={TaskIndex}
  Enable : Outport
  FinishIndex : Outport  Port=2
  wires:
  Switch Case/2 -> Subsystem/2(Case Default)
  Switch Case/1 -> Subsystem/1(Case)
  Subsystem/2(FinishIndex) -> FinishIndex/1
  Subsystem/1(Enable) -> Enable/1
  State/1 -> Switch Case/1

== system Robot/Motor3 Torque Control Init Frame/State_5_Enable ==
  State : Inport
  Subsystem : Subsystem
  Switch Case : SwitchCase  CaseConditions={TaskIndex}
  Enable : Outport
  FinishIndex : Outport  Port=2
  wires:
  Switch Case/2 -> Subsystem/2(Case Default)
  Switch Case/1 -> Subsystem/1(Case)
  Subsystem/2(FinishIndex) -> FinishIndex/1
  Subsystem/1(Enable) -> Enable/1
  State/1 -> Switch Case/1

== system Robot/Motor3 Torque Control Init Frame/State_6_Enable ==
  State : Inport
  Subsystem : Subsystem
  Switch Case : SwitchCase  CaseConditions={TaskIndex}
  Enable : Outport
  FinishIndex : Outport  Port=2
  wires:
  Switch Case/2 -> Subsystem/2(Case Default)
  Switch Case/1 -> Subsystem/1(Case)
  Subsystem/2(FinishIndex) -> FinishIndex/1
  Subsystem/1(Enable) -> Enable/1
  State/1 -> Switch Case/1

== system Robot/Motor3 Torque Control Init Frame/State_7_Enable ==
  State : Inport
  Subsystem : Subsystem
  Switch Case : SwitchCase  CaseConditions={TaskIndex}
  Enable : Outport
  FinishIndex : Outport  Port=2
  wires:
  Switch Case/2 -> Subsystem/2(Case Default)
  Switch Case/1 -> Subsystem/1(Case)
  Subsystem/2(FinishIndex) -> FinishIndex/1
  Subsystem/1(Enable) -> Enable/1
  State/1 -> Switch Case/1

== system Robot/Motor3 Torque Control Init Frame/State_8_Enable ==
  State : Inport
  Subsystem : Subsystem
  Switch Case : SwitchCase  CaseConditions={TaskIndex}
  Enable : Outport
  FinishIndex : Outport  Port=2
  wires:
  Switch Case/2 -> Subsystem/2(Case Default)
  Switch Case/1 -> Subsystem/1(Case)
  Subsystem/2(FinishIndex) -> FinishIndex/1
  Subsystem/1(Enable) -> Enable/1
  State/1 -> Switch Case/1

== system Robot/Motor3 Torque Control Init Frame/State_9_Enable ==
  State : Inport
  Subsystem : Subsystem
  Switch Case : SwitchCase  CaseConditions={TaskIndex}
  Enable : Outport
  FinishIndex : Outport  Port=2
  wires:
  Switch Case/2 -> Subsystem/2(Case Default)
  Switch Case/1 -> Subsystem/1(Case)
  Subsystem/2(FinishIndex) -> FinishIndex/1
  Subsystem/1(Enable) -> Enable/1
  State/1 -> Switch Case/1

== system Robot/Motor4 Torque Control Init Frame/Get MasterState OP Frame ==
  FinishIndex : Inport
  Enable : EnablePort
  Clock : Clock
  Constant4 : Constant  Value=0  OutDataTypeStr=double
  Constant5 : Constant
  Display{1,3..5} (4 alike) : Display
  EtherCAT PDO Receive1 : slrealtimeethercatlib/EtherCAT PDO Receive  Priority=2  sig_name=Drive 4 (Elmo Drive ).Inputs.Status word  sig_offset=39136  sig_type=uint16  type_size=16  sig_dim=1  device_id=0  sample_time=0.001000
  Get Device State : slrealtimeethercatlib/Get Device State  device_id=0  slave_name=Drive 4 (Elmo Drive )  sample_time=0.001  slave_addr=1004  selected_slave=Term 1 (EK1100)  timeout=500  slave_found=1
  If Action Subsystem5 : Subsystem  TreatAsAtomicUnit=on
  If Action Subsystem6 : Subsystem  TreatAsAtomicUnit=on
  If Action Subsystem7 : Subsystem  TreatAsAtomicUnit=on
  If1 : If  IfExpression=(u1 == 4663)
  If2 : If  IfExpression=(u1 == 8)
  Merge1 : Merge
  TaskFinished : Outport
  wires:
  If Action Subsystem6/1(Out1) -> Merge1/2
  EtherCAT PDO Receive1/1 -> Display3/1
  Get Device State/1 -> If2/1, Display1/1
  If Action Subsystem7/1(Out1) -> Display5/1
  If Action Subsystem5/1(Out1) -> Merge1/1
  Constant4/1 -> If Action Subsystem6/1(In1)
  Merge1/1 -> TaskFinished/1
  If1/1 -> If Action Subsystem7/Action
  Constant5/1 -> If Action Subsystem7/1(In1)
  If2/1 -> If Action Subsystem5/Action
  If2/2 -> If Action Subsystem6/Action
  Clock/1 -> Display4/1
  FinishIndex/1 -> If Action Subsystem5/1(In1)

== system Robot/Motor4 Torque Control Init Frame/PDO Set 0x6040:6->7->15 Frame ==
  FinishIndex : Inport
  Enable : EnablePort
  Clock : Clock
  Constant : Constant  Value=6  OutDataTypeStr=uint16
  Constant1 : Constant  Value=7  OutDataTypeStr=uint16
  Constant2 : Constant  Value=15  OutDataTypeStr=uint16
  Constant4 : Constant  Value=0  OutDataTypeStr=double
  Constant5 : Constant
  Counter Limited : simulink/Sources/Counter Limited  uplimit=500  tsamp=-1
  Display{1..5} (5 alike) : Display
  EtherCAT PDO Receive1 : slrealtimeethercatlib/EtherCAT PDO Receive  Priority=2  sig_name=Drive 4 (Elmo Drive ).Inputs.Status word  sig_offset=39136  sig_type=uint16  type_size=16  sig_dim=1  device_id=0  sample_time=0.001000
  EtherCAT PDO Transmit1 : slrealtimeethercatlib/EtherCAT PDO Transmit  Priority=3  sig_name=Drive 4 (Elmo Drive ).Outputs.Control word  sig_offset=39104  sig_type=uint16  type_size=16  sig_dim=1  device_id=0  sample_time=0.001000
  If : If  NumInputs=2  IfExpression=(u1 == 720)&(u2 == 500)  ElseIfExpressions=(u1 == 689)&(u2 == 500), (u1 == 691)&(u2 == 500)
  If Action Subsystem : Subsystem  TreatAsAtomicUnit=on
  If Action Subsystem1 : Subsystem  TreatAsAtomicUnit=on
  If Action Subsystem2 : Subsystem  TreatAsAtomicUnit=on
  If Action Subsystem4 : Subsystem  TreatAsAtomicUnit=on
  If Action Subsystem5 : Subsystem  TreatAsAtomicUnit=on
  If Action Subsystem6 : Subsystem  TreatAsAtomicUnit=on
  If Action Subsystem7 : Subsystem  TreatAsAtomicUnit=on
  If1 : If  IfExpression=(u1 == 4663)|(u1 == 4791)
  If2 : If  IfExpression=(u1 >= 0.1)
  Memory : Memory
  Merge : Merge  Inputs=4
  Merge1 : Merge
  TaskFinished : Outport
  wires:
  If Action Subsystem2/1(Out1) -> Merge/3
  If Action Subsystem7/1(Out1) -> If2/1, Display5/1
  If Action Subsystem6/1(Out1) -> Merge1/2
  EtherCAT PDO Receive1/1 -> If1/1, If/1, Display1/1
  If/2 -> If Action Subsystem1/Action
  Memory/1 -> If Action Subsystem4/1(In1)
  Constant5/1 -> If Action Subsystem7/1(In1)
  Constant1/1 -> If Action Subsystem1/1(In1)
  Constant/1 -> If Action Subsystem/1(In1)
  If Action Subsystem1/1(Out1) -> Merge/2
  If/4 -> If Action Subsystem4/Action
  Constant2/1 -> If Action Subsystem2/1(In1)
  If/3 -> If Action Subsystem2/Action
  If/1 -> If Action Subsystem/Action
  Clock/1 -> Display4/1
  If1/1 -> If Action Subsystem7/Action
  If2/1 -> If Action Subsystem5/Action
  Merge/1 -> Display2/1, EtherCAT PDO Transmit1/1, Memory/1
  Merge1/1 -> TaskFinished/1
  FinishIndex/1 -> If Action Subsystem5/1(In1)
  If2/2 -> If Action Subsystem6/Action
  If Action Subsystem4/1(Out1) -> Merge/4
  Counter Limited/1 -> If/2, Display3/1
  Constant4/1 -> If Action Subsystem6/1(In1)
  If Action Subsystem5/1(Out1) -> Merge1/1
  If Action Subsystem/1(Out1) -> Merge/1

== system Robot/Motor4 Torque Control Init Frame/SDO Get 0x6075 Frame ==
  FinishIndex : Inport
  Enable : EnablePort
  Clock : Clock
  Constant : Constant  OutDataTypeStr=int32
  Constant4 : Constant  Value=0  OutDataTypeStr=double
  Constant5 : Constant
  Display{,1,3..5} (5 alike) : Display
  EtherCAT Async SDO Upload : slrealtimeethercatlib/EtherCAT Async SDO Upload  index=0x6075  subIndex=0  sig_type=uint32  sig_dim=1  device_id=0  slave_name=Drive 4 (Elmo Drive )  sample_time=-1  slave_addr=1004  selected_slave=Term 1 (EK1100)  timeout=3000  slave_found=1  complete=0
  If Action Subsystem5 : Subsystem  TreatAsAtomicUnit=on
  If Action Subsystem6 : Subsystem  TreatAsAtomicUnit=on
  If Action Subsystem7 : Subsystem  TreatAsAtomicUnit=on
  If1 : If  IfExpression=(u1 == 4663)
  If2 : If  IfExpression=(u1 == 2)
  Merge1 : Merge
  TaskFinished : Outport
  RatedCurrent : Outport  Port=2
  wires:
  EtherCAT Async SDO Upload/1 -> RatedCurrent/1, Display/1
  EtherCAT Async SDO Upload/3 -> Display3/1
  EtherCAT Async SDO Upload/2 -> If2/1, Display1/1
  Constant/1 -> EtherCAT Async SDO Upload/1
  If2/1 -> If Action Subsystem5/Action
  Merge1/1 -> TaskFinished/1
  Clock/1 -> Display4/1
  If2/2 -> If Action Subsystem6/Action
  If Action Subsystem7/1(Out1) -> Display5/1
  Constant4/1 -> If Action Subsystem6/1(In1)
  If1/1 -> If Action Subsystem7/Action
  If Action Subsystem5/1(Out1) -> Merge1/1
  If Action Subsystem6/1(Out1) -> Merge1/2
  Constant5/1 -> If Action Subsystem7/1(In1)
  FinishIndex/1 -> If Action Subsystem5/1(In1)

== system Robot/Motor4 Torque Control Init Frame/SDO Set 0x6040:15 Frame ==
  FinishIndex : Inport
  Enable : EnablePort
  Bitwise Operator : simulink/Logic and Bit Operations/Bitwise Operator  logicop=AND  UseBitMask=on  BitMask=bin2dec('0000000000000111')  BitMaskRealWorld=Stored Integer
  Clock : Clock
  Constant : Constant  Value=15  OutDataTypeStr=uint16
  Constant1 : Constant  OutDataTypeStr=int32
  Constant2 : Constant  Value=0  OutDataTypeStr=int32
  Constant4 : Constant  Value=0  OutDataTypeStr=double
  Constant5 : Constant
  Constant6 : Constant  OutDataTypeStr=int32
  Constant7 : Constant
  Constant8 : Constant  Value=0b0000000000000111  OutDataTypeStr=uint16
  Display{1..6} (6 alike) : Display
  EtherCAT Async SDO Download : slrealtimeethercatlib/EtherCAT Async SDO Download  index=0x6040  subIndex=0  sig_type=uint16  sig_dim=1  device_id=0  slave_name=Drive 4 (Elmo Drive )  sample_time=-1  slave_addr=1004  selected_slave=Term 1 (EK1100)  timeout=2000  slave_found=1  complete=0
  EtherCAT PDO Receive1 : slrealtimeethercatlib/EtherCAT PDO Receive  Priority=2  sig_name=Drive 4 (Elmo Drive ).Inputs.Status word  sig_offset=39136  sig_type=uint16  type_size=16  sig_dim=1  device_id=0  sample_time=0.001
  If Action Subsystem1 : Subsystem  TreatAsAtomicUnit=on
  If Action Subsystem2 : Subsystem  TreatAsAtomicUnit=on
  If Action Subsystem3 : Subsystem  TreatAsAtomicUnit=on
  If Action Subsystem5 : Subsystem  TreatAsAtomicUnit=on
  If Action Subsystem6 : Subsystem  TreatAsAtomicUnit=on
  If Action Subsystem7 : Subsystem  TreatAsAtomicUnit=on
  If1 : If  IfExpression=(u1 == 4663)
  If2 : If  IfExpression=(u1 == 2)
  If3 : If  NumInputs=2  IfExpression=(u1 == u2)
  If4 : If  IfExpression=(u1 >= 0.1)
  Merge1 : Merge
  Merge2 : Merge
  TaskFinished : Outport
  wires:
  Constant8/1 -> If3/2
  Bitwise Operator/1 -> If3/1
  If Action Subsystem3/1(Out1) -> Display6/1, If4/1
  Clock/1 -> Display4/1
  Merge1/1 -> TaskFinished/1
  If Action Subsystem2/1(Out1) -> Merge2/2
  If Action Subsystem1/1(Out1) -> Merge2/1
  Constant7/1 -> If Action Subsystem3/1(In1)
  If2/2 -> If Action Subsystem6/Action
  EtherCAT PDO Receive1/1 -> Display3/1, Bitwise Operator/1
  If3/1 -> If Action Subsystem3/Action
  If4/1 -> If Action Subsystem1/Action
  Constant6/1 -> If Action Subsystem2/1(In1)
  If4/2 -> If Action Subsystem2/Action
  EtherCAT Async SDO Download/1 -> If2/1, Display1/1
  Constant4/1 -> If Action Subsystem6/1(In1)
  Constant5/1 -> If Action Subsystem7/1(In1)
  Constant1/1 -> EtherCAT Async SDO Download/2
  If Action Subsystem6/1(Out1) -> Merge1/2
  If Action Subsystem7/1(Out1) -> Display5/1
  If2/1 -> If Action Subsystem5/Action
  Constant2/1 -> If Action Subsystem1/1(In1)
  If1/1 -> If Action Subsystem7/Action
  FinishIndex/1 -> If Action Subsystem5/1(In1)
  EtherCAT Async SDO Download/2 -> Display2/1
  Constant/1 -> EtherCAT Async SDO Download/1
  If Action Subsystem5/1(Out1) -> Merge1/1

== system Robot/Motor4 Torque Control Init Frame/SDO Set 0x6040:31 Frame ==
  FinishIndex : Inport
  Enable : EnablePort
  Bitwise Operator : simulink/Logic and Bit Operations/Bitwise Operator  logicop=AND  UseBitMask=on  BitMask=bin2dec('0001010000010111')  BitMaskRealWorld=Stored Integer
  Clock : Clock
  Constant : Constant  Value=31  OutDataTypeStr=uint16
  Constant1 : Constant  OutDataTypeStr=int32
  Constant2 : Constant  Value=0  OutDataTypeStr=int32
  Constant4 : Constant  Value=0  OutDataTypeStr=double
  Constant5 : Constant
  Constant6 : Constant  OutDataTypeStr=int32
  Constant7 : Constant
  Constant8 : Constant  Value=0b0001010000010111  OutDataTypeStr=uint16
  Display{1..6} (6 alike) : Display
  EtherCAT Async SDO Download : slrealtimeethercatlib/EtherCAT Async SDO Download  index=0x6040  subIndex=0  sig_type=uint16  sig_dim=1  device_id=0  slave_name=Drive 4 (Elmo Drive )  sample_time=-1  slave_addr=1004  selected_slave=Term 1 (EK1100)  timeout=2000  slave_found=1  complete=0
  EtherCAT PDO Receive1 : slrealtimeethercatlib/EtherCAT PDO Receive  Priority=2  sig_name=Drive 4 (Elmo Drive ).Inputs.Status word  sig_offset=39136  sig_type=uint16  type_size=16  sig_dim=1  device_id=0  sample_time=0.001
  If Action Subsystem1 : Subsystem  TreatAsAtomicUnit=on
  If Action Subsystem2 : Subsystem  TreatAsAtomicUnit=on
  If Action Subsystem3 : Subsystem  TreatAsAtomicUnit=on
  If Action Subsystem5 : Subsystem  TreatAsAtomicUnit=on
  If Action Subsystem6 : Subsystem  TreatAsAtomicUnit=on
  If Action Subsystem7 : Subsystem  TreatAsAtomicUnit=on
  If1 : If  IfExpression=(u1 == 4663)
  If2 : If  IfExpression=(u1 == 2)
  If3 : If  NumInputs=2  IfExpression=(u1 == u2)
  If4 : If  IfExpression=(u1 >= 0.1)
  Merge1 : Merge
  Merge2 : Merge
  TaskFinished : Outport
  wires:
  If1/1 -> If Action Subsystem7/Action
  If Action Subsystem5/1(Out1) -> Merge1/1
  If Action Subsystem6/1(Out1) -> Merge1/2
  FinishIndex/1 -> If Action Subsystem5/1(In1)
  If2/1 -> If Action Subsystem5/Action
  If4/2 -> If Action Subsystem2/Action
  EtherCAT Async SDO Download/1 -> If2/1, Display1/1
  Constant/1 -> EtherCAT Async SDO Download/1
  Bitwise Operator/1 -> If3/1
  If Action Subsystem7/1(Out1) -> Display5/1
  Constant8/1 -> If3/2
  If2/2 -> If Action Subsystem6/Action
  If Action Subsystem3/1(Out1) -> Display6/1, If4/1
  If Action Subsystem2/1(Out1) -> Merge2/2
  If3/1 -> If Action Subsystem3/Action
  Constant4/1 -> If Action Subsystem6/1(In1)
  Constant6/1 -> If Action Subsystem2/1(In1)
  If4/1 -> If Action Subsystem1/Action
  Constant1/1 -> EtherCAT Async SDO Download/2
  EtherCAT PDO Receive1/1 -> Display3/1, Bitwise Operator/1
  Clock/1 -> Display4/1
  If Action Subsystem1/1(Out1) -> Merge2/1
  Merge1/1 -> TaskFinished/1
  Constant2/1 -> If Action Subsystem1/1(In1)
  EtherCAT Async SDO Download/2 -> Display2/1
  Constant5/1 -> If Action Subsystem7/1(In1)
  Constant7/1 -> If Action Subsystem3/1(In1)
